simulink model "Requirements"  (R2020a)
settings: Solver=FixedStepAuto  StartTime=0.0  StopTime=10.0  RelTol=1e-3
undefined symbols (not defined in the file): DiscIntNeverNeededParam, sldvsubsys
libraries: sldvlib x6
settings Model: Creator=vivek vivian  LastModifiedBy=vivek vivian
settings ConfigComp: DVMode=PropertyProving  DVMaxProcessTime=NaN  DVTestSuiteOptimization=Auto  DVDetectOutOfBounds=on

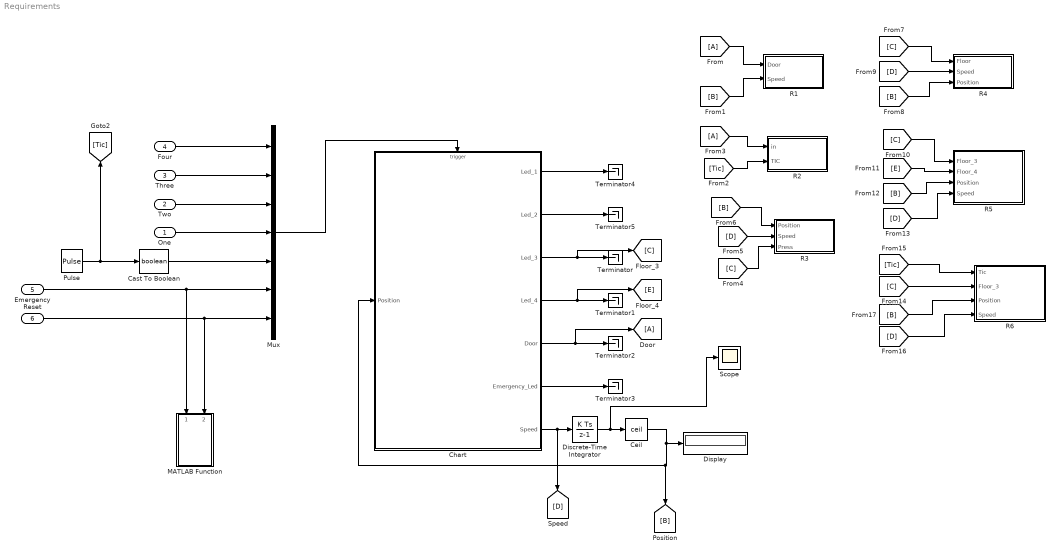
== system Requirements ==
  One : Inport  OutDataTypeStr=boolean
  Two : Inport  Port=2  OutDataTypeStr=boolean
  Three : Inport  Port=3  OutDataTypeStr=boolean
  Four : Inport  Port=4  OutDataTypeStr=boolean
  Emergency : Inport  Port=5  OutDataTypeStr=boolean
  Reset : Inport  Port=6  OutDataTypeStr=boolean
  Cast To Boolean : DataTypeConversion  OutDataTypeStr=boolean
  Ceil : Rounding  Operator=ceil
  Chart : Stateflow chart  TreatAsAtomicUnit=on
  Discrete-Time Integrator : DiscreteIntegrator  InitialCondition=0.01  SampleTime=-1  ICPrevOutput=DiscIntNeverNeededParam  ICPrevScaledInput=DiscIntNeverNeededParam
  Display : Display
  MATLAB Function : MATLAB Function  TreatAsAtomicUnit=on
  Mux : Mux  Inputs=7
  Pulse : DiscretePulseGenerator  PulseType=Time based  Period=1  PulseWidth=5
  R1 : Subsystem  Tag=VerificationSubsystem  DisableCoverage=on  LoadFcn=sldvsubsys('check')  TreatAsAtomicUnit=on  SimViewingDevice=on  mask(VerificationSubsystem){}
      mask init:
      | sldvsubsys('maskInit');
      settings: CopyFcn=sldvsubsys('copy');  OpenFcn=open_system(gcb,'force');
      settings: PreSaveFcn=|
      | set_param(gcb,'SimViewingDevice','on');
      | sldvsubsys('check');
      mask Help: helpview(fullfile(docroot,'toolbox','sldv','sldv.map'),'verificationsubsystem')
      mask Display: image(imread('sldvicon_versubsys.png','BackGroundColor',[1 1 1]),'center');
  R2 : Subsystem  Tag=VerificationSubsystem  DisableCoverage=on  LoadFcn=sldvsubsys('check')  TreatAsAtomicUnit=on  SimViewingDevice=on  mask(VerificationSubsystem){}
      mask init:
      | sldvsubsys('maskInit');
      settings: CopyFcn=sldvsubsys('copy');  OpenFcn=open_system(gcb,'force');
      settings: PreSaveFcn=|
      | set_param(gcb,'SimViewingDevice','on');
      | sldvsubsys('check');
      mask Help: helpview(fullfile(docroot,'toolbox','sldv','sldv.map'),'verificationsubsystem')
      mask Display: image(imread('sldvicon_versubsys.png','BackGroundColor',[1 1 1]),'center');
  R3 : Subsystem  Tag=VerificationSubsystem  DisableCoverage=on  LoadFcn=sldvsubsys('check')  TreatAsAtomicUnit=on  SimViewingDevice=on  mask(VerificationSubsystem){}
      mask init:
      | sldvsubsys('maskInit');
      settings: CopyFcn=sldvsubsys('copy');  OpenFcn=open_system(gcb,'force');
      settings: PreSaveFcn=|
      | set_param(gcb,'SimViewingDevice','on');
      | sldvsubsys('check');
      mask Help: helpview(fullfile(docroot,'toolbox','sldv','sldv.map'),'verificationsubsystem')
      mask Display: image(imread('sldvicon_versubsys.png','BackGroundColor',[1 1 1]),'center');
  R4 : Subsystem  Tag=VerificationSubsystem  DisableCoverage=on  LoadFcn=sldvsubsys('check')  TreatAsAtomicUnit=on  SimViewingDevice=on  mask(VerificationSubsystem){}
      mask init:
      | sldvsubsys('maskInit');
      settings: CopyFcn=sldvsubsys('copy');  OpenFcn=open_system(gcb,'force');
      settings: PreSaveFcn=|
      | set_param(gcb,'SimViewingDevice','on');
      | sldvsubsys('check');
      mask Help: helpview(fullfile(docroot,'toolbox','sldv','sldv.map'),'verificationsubsystem')
      mask Display: image(imread('sldvicon_versubsys.png','BackGroundColor',[1 1 1]),'center');
  R5 : Subsystem  Tag=VerificationSubsystem  DisableCoverage=on  LoadFcn=sldvsubsys('check')  TreatAsAtomicUnit=on  SimViewingDevice=on  mask(VerificationSubsystem){}
      mask init:
      | sldvsubsys('maskInit');
      settings: CopyFcn=sldvsubsys('copy');  OpenFcn=open_system(gcb,'force');
      settings: PreSaveFcn=|
      | set_param(gcb,'SimViewingDevice','on');
      | sldvsubsys('check');
      mask Help: helpview(fullfile(docroot,'toolbox','sldv','sldv.map'),'verificationsubsystem')
      mask Display: image(imread('sldvicon_versubsys.png','BackGroundColor',[1 1 1]),'center');
  R6 : Subsystem
  Scope : Scope
  Terminator{,1..5} (6 alike) : Terminator
  wires:
  Two/1 -> Mux/3
  Emergency/1 -> MATLAB Function/1(Emergency), Mux/6
  One/1 -> Mux/4
  [C] -> R3/3(Press)
  Four/1 -> Mux/1
  Chart/7(Speed) -> Discrete-Time Integrator/1, [D]
  Three/1 -> Mux/2
  Discrete-Time Integrator/1 -> Scope/1, Ceil/1
  Chart/3(Led_3) -> [C], Terminator/1
  [Tic] -> R2/2(TIC)
  Chart/1(Led_1) -> Terminator4/1
  [A] -> R1/1(Door)
  Pulse/1 -> Cast To Boolean/1, [Tic]
  [A] -> R2/1(in)
  [B] -> R1/2(Speed)
  Chart/2(Led_2) -> Terminator5/1
  [B] -> R3/1(Position)
  [D] -> R3/2(Speed)
  Cast To Boolean/1 -> Mux/5
  Ceil/1 -> Chart/1(Position), [B], Display/1
  Chart/4(Led_4) -> [E], Terminator1/1
  Chart/5(Door) -> [A], Terminator2/1
  Mux/1 -> Chart/Trigger
  Reset/1 -> MATLAB Function/2(Reset), Mux/7
  Chart/6(Emergency_Led) -> Terminator3/1
  [C] -> R4/1(Floor)
  [D] -> R4/2(Speed)
  [B] -> R4/3(Position)
  [E] -> R5/2(Floor_4)
  [C] -> R5/1(Floor_3)
  [B] -> R5/3(Position)
  [D] -> R5/4(Speed)
  [Tic] -> R6/1(Tic)
  [C] -> R6/2(Floor_3)
  [B] -> R6/3(Position)
  [D] -> R6/4(Speed)

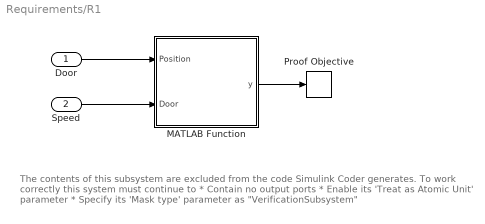
== system Requirements/R1 ==
  note: The contents of this subsystem are excluded from the code Simulink Coder
      | generates.
      |
      | To work correctly this system must continue to
      | * Contain no output ports
      | * Enable its 'Treat as Atomic Unit' parameter
      | * Specify its 'Mask type' parameter as "VerificationSubsystem"
  Door : Inport
  Speed : Inport  Port=2
  MATLAB Function : MATLAB Function  TreatAsAtomicUnit=on
  Proof Objective : sldvlib/Objectives and Constraints/Proof Objective  enabled=on  customAVTBlockType=Proof Objective  intervals=true  dispValues=on  outEnabled=off  enableStopSim=off
      settings: AttributesFormatString=%<intervals>  SourceProductBaseCode=SL
  wires:
  Speed/1 -> MATLAB Function/2(Door)
  MATLAB Function/1(y) -> Proof Objective/1
  Door/1 -> MATLAB Function/1(Position)

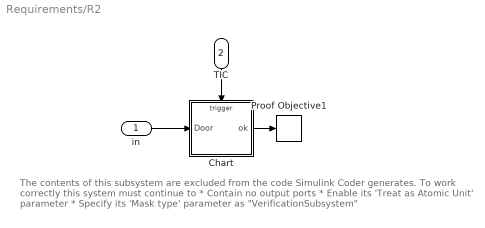
== system Requirements/R2 ==
  note: The contents of this subsystem are excluded from the code Simulink Coder
      | generates.
      |
      | To work correctly this system must continue to
      | * Contain no output ports
      | * Enable its 'Treat as Atomic Unit' parameter
      | * Specify its 'Mask type' parameter as "VerificationSubsystem"
  in : Inport
  TIC : Inport  Port=2
  Chart : Stateflow chart  TreatAsAtomicUnit=on
  Proof Objective1 : sldvlib/Objectives and Constraints/Proof Objective  enabled=on  customAVTBlockType=Proof Objective  intervals=false  dispValues=on  outEnabled=off  enableStopSim=off
      settings: AttributesFormatString=%<intervals>  SourceProductBaseCode=SL
  wires:
  in/1 -> Chart/1(Door)
  TIC/1 -> Chart/Trigger
  Chart/1(ok) -> Proof Objective1/1

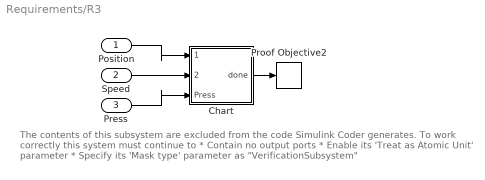
== system Requirements/R3 ==
  note: The contents of this subsystem are excluded from the code Simulink Coder
      | generates.
      |
      | To work correctly this system must continue to
      | * Contain no output ports
      | * Enable its 'Treat as Atomic Unit' parameter
      | * Specify its 'Mask type' parameter as "VerificationSubsystem"
  Position : Inport
  Speed : Inport  Port=2
  Press : Inport  Port=3
  Chart : Stateflow chart  TreatAsAtomicUnit=on
  Proof Objective2 : sldvlib/Objectives and Constraints/Proof Objective  enabled=on  customAVTBlockType=Proof Objective  intervals=false  dispValues=on  outEnabled=off  enableStopSim=off
      settings: AttributesFormatString=%<intervals>  SourceProductBaseCode=SL
  wires:
  Position/1 -> Chart/1(Position)
  Speed/1 -> Chart/2(Speed)
  Press/1 -> Chart/3(Press)
  Chart/1(done) -> Proof Objective2/1

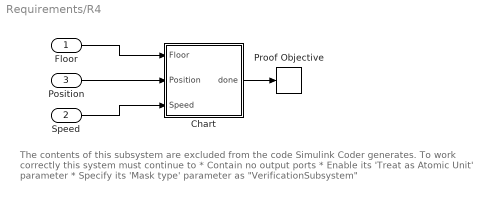
== system Requirements/R4 ==
  note: The contents of this subsystem are excluded from the code Simulink Coder
      | generates.
      |
      | To work correctly this system must continue to
      | * Contain no output ports
      | * Enable its 'Treat as Atomic Unit' parameter
      | * Specify its 'Mask type' parameter as "VerificationSubsystem"
  Floor : Inport
  Speed : Inport  Port=2
  Position : Inport  Port=3
  Chart : Stateflow chart  TreatAsAtomicUnit=on
  Proof Objective : sldvlib/Objectives and Constraints/Proof Objective  enabled=on  customAVTBlockType=Proof Objective  intervals=false  dispValues=on  outEnabled=off  enableStopSim=off
      settings: AttributesFormatString=%<intervals>  SourceProductBaseCode=SL
  wires:
  Floor/1 -> Chart/1(Floor)
  Speed/1 -> Chart/3(Speed)
  Position/1 -> Chart/2(Position)
  Chart/1(done) -> Proof Objective/1

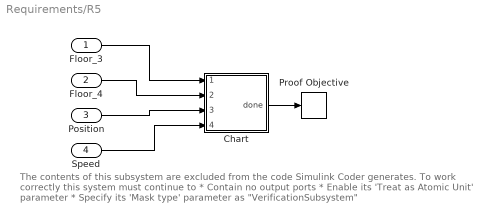
== system Requirements/R5 ==
  note: The contents of this subsystem are excluded from the code Simulink Coder
      | generates.
      |
      | To work correctly this system must continue to
      | * Contain no output ports
      | * Enable its 'Treat as Atomic Unit' parameter
      | * Specify its 'Mask type' parameter as "VerificationSubsystem"
  Floor_3 : Inport
  Floor_4 : Inport  Port=2
  Position : Inport  Port=3
  Speed : Inport  Port=4
  Chart : Stateflow chart  TreatAsAtomicUnit=on
  Proof Objective : sldvlib/Objectives and Constraints/Proof Objective  enabled=on  customAVTBlockType=Proof Objective  intervals=false  dispValues=on  outEnabled=off  enableStopSim=off
      settings: AttributesFormatString=%<intervals>  SourceProductBaseCode=SL
  wires:
  Floor_3/1 -> Chart/1(Floor_3)
  Floor_4/1 -> Chart/2(Floor_4)
  Position/1 -> Chart/3(Position)
  Speed/1 -> Chart/4(Speed)
  Chart/1(done) -> Proof Objective/1

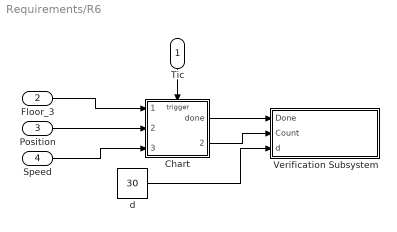
== system Requirements/R6 ==
  Tic : Inport
  Floor_3 : Inport  Port=2
  Position : Inport  Port=3
  Speed : Inport  Port=4
  Chart : Stateflow chart  TreatAsAtomicUnit=on
  Verification Subsystem : Subsystem  Tag=VerificationSubsystem  DisableCoverage=on  LoadFcn=sldvsubsys('check')  TreatAsAtomicUnit=on  SimViewingDevice=on  mask(VerificationSubsystem){}
      mask init:
      | sldvsubsys('maskInit');
      settings: CopyFcn=sldvsubsys('copy');  OpenFcn=open_system(gcb,'force');
      settings: PreSaveFcn=|
      | set_param(gcb,'SimViewingDevice','on');
      | sldvsubsys('check');
      mask Help: helpview(fullfile(docroot,'toolbox','sldv','sldv.map'),'verificationsubsystem')
      mask Display: image(imread('sldvicon_versubsys.png','BackGroundColor',[1 1 1]),'center');
  d : Constant  Value=30
  wires:
  Chart/2(count) -> Verification Subsystem/2(Count)
  d/1 -> Verification Subsystem/3(d)
  Chart/1(done) -> Verification Subsystem/1(Done)
  Position/1 -> Chart/2(Position)
  Speed/1 -> Chart/3(Speed)
  Tic/1 -> Chart/Trigger
  Floor_3/1 -> Chart/1(Floor_3)

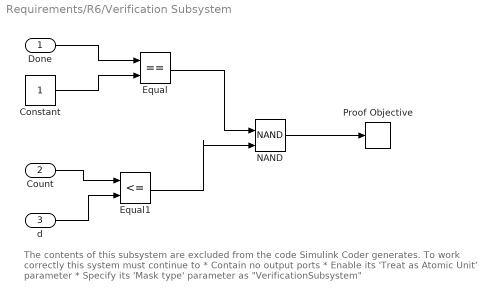
== system Requirements/R6/Verification Subsystem ==
  note: The contents of this subsystem are excluded from the code Simulink Coder
      | generates.
      |
      | To work correctly this system must continue to
      | * Contain no output ports
      | * Enable its 'Treat as Atomic Unit' parameter
      | * Specify its 'Mask type' parameter as "VerificationSubsystem"
  Done : Inport
  Count : Inport  Port=2
  d : Inport  Port=3
  Constant : Constant
  Equal : RelationalOperator  Operator===  OutDataTypeStr=boolean  RndMeth=Simplest
  Equal1 : RelationalOperator  Operator=<=  OutDataTypeStr=boolean  RndMeth=Simplest
  NAND : Logic  Operator=NAND  IconShape=distinctive  AllPortsSameDT=off  OutDataTypeStr=boolean
  Proof Objective : sldvlib/Objectives and Constraints/Proof Objective  enabled=on  customAVTBlockType=Proof Objective  intervals=true  dispValues=on  outEnabled=off  enableStopSim=off
      settings: AttributesFormatString=%<intervals>  SourceProductBaseCode=SL
  wires:
  Done/1 -> Equal/1
  Constant/1 -> Equal/2
  Count/1 -> Equal1/1
  d/1 -> Equal1/2
  Equal/1 -> NAND/1
  Equal1/1 -> NAND/2
  NAND/1 -> Proof Objective/1

== stateflow chart Requirements/R4/Chart ==
  state Initial
  state is_Press
  state Bad
    en:done=1;
  state is_stopped
  state pressed
  (default) -> Initial : {done=0;}
  pressed -> Initial [order 2] : [Position ~= 3 && Speed~=0]
  Initial -> is_Press : [Floor==1]
  pressed -> Bad [order 1] : [Position == 3 && Speed==0]
  is_Press -> is_stopped : [Position==3&&Speed==0]
  is_stopped -> pressed : [Position ~= 3 && Speed~=0]
  data: Floor input; Position input; Speed input; done output

== stateflow chart Requirements/R2/Chart ==
  state Init
    en:ok=0;
  state is_closed
  state is_open
  state error
    en:ok=1;
  (default) -> Init
  Init -> is_closed : [Door==0]
  is_closed -> is_open : [Door==1]
  is_open -> is_closed [order 1] : after(5,TIC)[Door==0]
  is_open -> error [order 2] : before(5,TIC)[Door==0]
  data: Door input; ok output
  events: TIC input RISING_EDGE_EVENT

== stateflow chart Requirements/Chart ==
  settings: executeAtInitialization=1
  state Emergency_State
    en: Speed=0;Emergency_Led=1;
  state Initial
    en:init();
  state Controller
    on One: queue(1) = 1;Led_1 = 1;
    on Two: queue(2) = 1;Led_2 = 1;
    on Three: queue(3) = 1;Led_3 =1;
    on Four: queue(4) = 1;Led_4 = 1;
    state Idle
      en: Direction = 0;
    state UP
      en: Direction=1;
      du:Speed = 0.2;
    state DOWN
      en: Direction=-1;
      du: Speed =-0.2;
    state Check_Down
      en:Speed=0;
    state Check_Up
      en:Speed=0;
    state Door
      en: Door=1;
      du: queue(Position) = 0;
    (default) -> Idle : {Door=0;led();}
    Idle -> DOWN [order 2] : [down==1]
    Idle -> UP [order 1] : [up==1]
    Idle -> Door [order 3] : [queue(Position)==1]
    (junction 528) -> Idle [order 3] : [none == 1]
    (junction 528) -> UP [order 1] : [up==1&&(Direction == 1||down==0)]
    (junction 528) -> DOWN [order 2] : [down==1&&up==0]
    DOWN -> Check_Down : [queue(Position)==1]
        | {led();}
    UP -> Check_Up : [queue(Position)==1]
        | {led();}
    Door -> (junction 528) : after(5,sec){Door=0;led();}
    Check_Up -> Door
    Check_Down -> Door
  (default) -> Initial
  Emergency_State -> Controller : Reset{Emergency_Led=0}
  Controller -> Emergency_State : Emergency
  Initial -> Controller
  data: y function_output; y function_output; y function_output; queue local double size=[1 4]; Led_1 output; Led_2 output; Led_3 output; Led_4 output; Door output; Emergency_Led output; Direction local; Speed output; destination local; Position input
  events: Four input RISING_EDGE_EVENT; Three input RISING_EDGE_EVENT; Two input RISING_EDGE_EVENT; One input RISING_EDGE_EVENT; TIC input RISING_EDGE_EVENT; Emergency input RISING_EDGE_EVENT; Reset input RISING_EDGE_EVENT
  function init:
    | function init()
    | Led_1=0;
    | Led_2=0;
    | Led_3=0;
    | Led_4=0;
    | Door=0;
    | Emergency_Led=0;
    | queue=[0 0 0 0];
    | destination=0;
    | end
  function y = down:
    | function y = down
    | y=0;
    | if queue(1) == 1 
    |     destination = 1;
    |     if Position < destination 
    |         y = 0;
    |     elseif Position > destination
    |         y = 1;
    |     end
    | elseif queue(2) == 1 
    |     destination = 2;
    |     if Position < destination 
    |         y = 0;
    |     elseif Position > destination
    |         y = 1;
    |     end
    | elseif queue(3) == 1 
    |     destination = 3;
    |    if Position < destination 
    |         y = 0;
    |     elseif Position > destination
    |         y = 1;
    |     end
    | elseif queue(4) == 1 
    |     destination = 4;
    |     if Position < destination 
    |         y = 0;
    |     elseif Position > destination
    |         y = 1;
    |     end
    | end
    | end
  function led:
    | function led
    | if Position == 1 && Led_1 == 1
    |     Led_1 = 0;
    | elseif Position == 2 && Led_2 == 1
    |     Led_2 = 0;
    | elseif Position == 3 && Led_3 == 1
    |     Led_3 = 0;
    | elseif Position == 4 && Led_4 == 1
    |     Led_4 = 0;
    | else
    | end
  function y = up:
    | function y = up
    | y=0;
    | if queue(4) == 1 
    |     destination = 4;
    |     if Position < destination 
    |         y = 1;
    |     elseif Position > destination
    |         y = 0;
    |     end
    | elseif queue(3) == 1 
    |     destination = 3;
    |    if Position < destination
    |         y = 1;
    |     elseif Position > destination
    |         y = 0;
    |    end
    | elseif queue(2) == 1 
    |     destination = 2;
    |     if Position < destination 
    |         y = 1;
    |     elseif Position > destination
    |         y = 0;
    |     end
    | elseif queue(1) == 1 
    |     destination = 1;
    |     if Position < destination 
    |         y = 1;
    |     elseif Position > destination
    |         y = 0;
    |     end
    | end
    | end
  function y = none:
    | function y = none
    | if queue(1) == 0 && queue(2) == 0 && queue(3) == 0 && queue(4) == 0 
    |     y = 1;
    | else
    |     y = 0;
    | end

== matlab function Requirements/R1/MATLAB Function ==
  data: Position input; y output; Door input
function y = fcn(Position,Door)
if (Position ~= 1 || Position ~= 2 || Position ~= 3 || Position ~= 4)&& (Door==1)
    y = true;
else
    y = false;
end

== stateflow chart Requirements/R3/Chart ==
  state initial
    en:done=0;
  state Floor
  state Check
  (default) -> initial
  initial -> Check [order 2] : [Position==3&&Speed==0]{done=1;}
  initial -> Floor [order 1] : [Press == 1]
  Floor -> Check : [Position==3&&Speed==0]
  data: Position input; Speed input; done output; Press input

== matlab function Requirements/MATLAB Function ==
  data: Emergency input; Reset input
function fcn(Emergency,Reset)
sldv.assume(Emergency+Reset ==0);
end

== stateflow chart Requirements/R5/Chart ==
  state Bad
  state Initial
  state Unsatisfied
    en:done=1;
  state is_pressed1
  state is_pressed
  state Reach_4
  state Again
  state Reach_3
  (default) -> Initial : {done=0;}
  Bad -> Unsatisfied : [Position==3&&Speed==0]
  is_pressed -> Bad [order 2] : [Floor_3==1&&Position>3]
  Initial -> is_pressed : [Floor_4==1]
  is_pressed -> is_pressed1 [order 1] : [Floor_3==1&&Position<=3]
  is_pressed1 -> Reach_3 : [Position==3&&Speed==0]
  is_pressed -> Reach_4 [order 3] : [Position==4&&Speed==0]
  Again -> Reach_3 [order 1] : [Position==3&&Speed==0]{done=1;}
  Again -> Reach_4 [order 2] : [Position==4&&Speed==0]
  Reach_3 -> Again : [Position~=3&&Speed~=0]
  data: Floor_3 input; Floor_4 input; Position input; Speed input; done output

== stateflow chart Requirements/R6/Chart ==
  state Initial
    en:count=0;
  state Is_pressed
    on TIC: count=count+1;
  state Reached_3
    en:done=1;
  (default) -> Initial : {done=0;}
  Initial -> Is_pressed : [Floor_3==1]
  Is_pressed -> Reached_3 : [Position==3&&Speed==0]
  data: Floor_3 input; Position input; Speed input; done output; count output
  events: TIC input RISING_EDGE_EVENT
